simulink model "iddemsl3"  (Simulink 3.00)
settings: Solver=ode45  StartTime=0.0  StopTime=500  RelTol=1e-3
libraries: simulink3 x1
settings Model: IntegerOverflowMsg=none

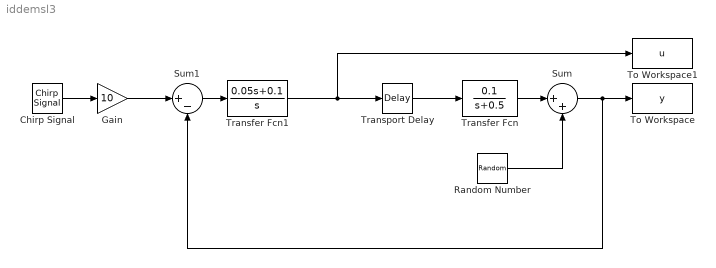
== system iddemsl3 ==
  Chirp Signal : simulink3/Sources/Chirp Signal  f1=0.001  T=500  f2=0.7
  Gain : Gain  Gain=10  SaturateOnIntegerOverflow=on
  Random Number : RandomNumber  Mean=0  Variance=0.01  Seed=0  SampleTime=0.5
  Sum : Sum  Inputs=|++  SaturateOnIntegerOverflow=on
  Sum1 : Sum  Inputs=|+-  SaturateOnIntegerOverflow=on
  To Workspace : ToWorkspace  VariableName=y  SampleTime=0.5  SaveFormat=Matrix
  To Workspace1 : ToWorkspace  VariableName=u  SampleTime=0.5  SaveFormat=Matrix
  Transfer Fcn : TransferFcn  Numerator=0.1  Denominator=[1 0.5]
  Transfer Fcn1 : TransferFcn  Numerator=[0.05 0.1]  Denominator=[1 0]
  Transport Delay : TransportDelay  DelayTime=1.001  InitialInput=0  BufferSize=1024
  wires:
  Transport Delay/1 -> Transfer Fcn/1
  Transfer Fcn/1 -> Sum/1
  Random Number/1 -> Sum/2
  Sum1/1 -> Transfer Fcn1/1
  Sum/1 -> To Workspace/1, Sum1/2
  Chirp Signal/1 -> Gain/1
  Gain/1 -> Sum1/1
  Transfer Fcn1/1 -> Transport Delay/1, To Workspace1/1
